simulink model "position_lqi_controller_double_loop_sim"  (R2023b)
settings: Solver=ode4  StartTime=0.0  StopTime=5  FixedStep=0.001  RelTol=1e-3  EnableMultiTasking=on
undefined symbols (not defined in the file or in its folder): K
libraries: simulink_extras x2, cstblocks x1
settings Model: ExtModeTrigDuration=10  Creator=paoli  LastModifiedBy=paoli
settings OptimizationCC: DefaultParameterBehavior=Inlined  EnhancedBackFolding=on  PassReuseOutputArgsAs=Individual arguments  ZeroExternalMemoryAtStartup=off  ZeroInternalMemoryAtStartup=off  MaxStackSize=64  OptimizeBlockOrder=speed  DifferentSizesBufferReuse=on  OptimizationCustomize=off  EfficientTunableParamExpr=on
settings DebuggingCC: ParameterTunabilityLossMsg=error
settings HardwareCC: ProdBitPerPointer=32  ProdBitPerSizeT=32  ProdBitPerPtrDiffT=32  ProdLargestAtomicInteger=Long  ProdLargestAtomicFloat=Double  ProdWordSize=32  ProdLongLongMode=on  ProdHWDeviceType=ARM Compatible->ARM Cortex
settings SFSimCC: MATLABDynamicMemAlloc=off
settings RTWCC: Description=Embedded Coder  SystemTargetFile=ert.tlc  TemplateMakefile=ert_default_tmf  Toolchain=GNU Tools for ARM Embedded Processors
settings CodeAppCC: ForceParamTrailComments=on  IgnoreCustomStorageClasses=off  OperatorAnnotations=on  SimulinkDataObjDesc=on  SFDataObjDesc=on  InsertBlockDesc=on
settings ERTTargetCC: SupportContinuousTime=on  ExtModeTransport=3  ExtModeStaticAlloc=on  ExtModeStaticAllocSize=2000  ExtModeMexFile=ext_xcp  ExtModeIntrfLevel=Level2 - Open  InlinedParameterPlacement=NonHierarchical  ERTCustomFileTemplate=example_file_process.tlc

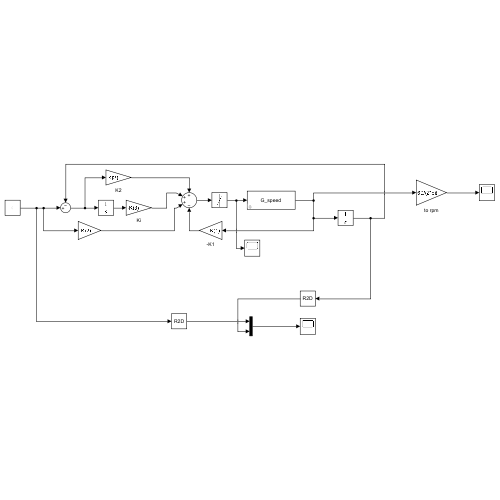
[thumbnail: Simulink's stored preview of the top-level diagram]
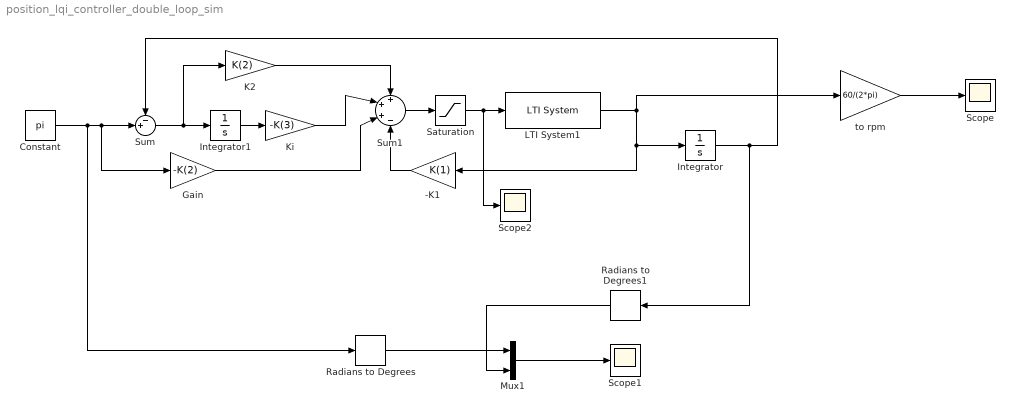
== system position_lqi_controller_double_loop_sim ==
  -K1 : Gain  Gain=K(1)
  Constant : Constant  Value=pi
  Gain : Gain  Gain=-K(2)
  Integrator : Integrator
  Integrator1 : Integrator
  K2 : Gain  Gain=K(2)
  Ki : Gain  Gain=-K(3)
  LTI System1 : cstblocks/LTI System  sys=G_speed  IC=[]  PadeOrder=0
  Mux1 : Mux  Inputs=2
  Radians to Degrees : simulink_extras/Transformations/Radians to Degrees
  Radians to Degrees1 : simulink_extras/Transformations/Radians to Degrees
  Saturation : Saturate  UpperLimit=12  LowerLimit=-12
  Scope : Scope
  Scope1 : Scope
  Scope2 : Scope
  Sum : Sum  Inputs=-+|
  Sum1 : Sum  Inputs=+++-
  to rpm : Gain  Gain=60/(2*pi)
  wires:
  Integrator/1 -> Sum/1, Radians to Degrees1/1
  to rpm/1 -> Scope/1
  Constant/1 -> Gain/1, Sum/2, Radians to Degrees/1
  Mux1/1 -> Scope1/1
  Sum1/1 -> Saturation/1
  Saturation/1 -> Scope2/1, LTI System1/1
  Radians to Degrees/1 -> Mux1/1
  Radians to Degrees1/1 -> Mux1/2
  -K1/1 -> Sum1/4
  K2/1 -> Sum1/1
  Ki/1 -> Sum1/2
  Integrator1/1 -> Ki/1
  Sum/1 -> K2/1, Integrator1/1
  LTI System1/1 -> -K1/1, Integrator/1, to rpm/1
  Gain/1 -> Sum1/3
